simulink model "thesis_DLF_V1"  (R2024b)
settings: Solver=VariableStepAuto  StartTime=0.0  StopTime=40  FixedStep=0.001  RelTol=1e-3  EnableMultiTasking=on
undefined symbols (not defined in the file or in its folder): omega_0, p0, R0, v0
settings Model: Creator=bojack  LastModifiedBy=valer

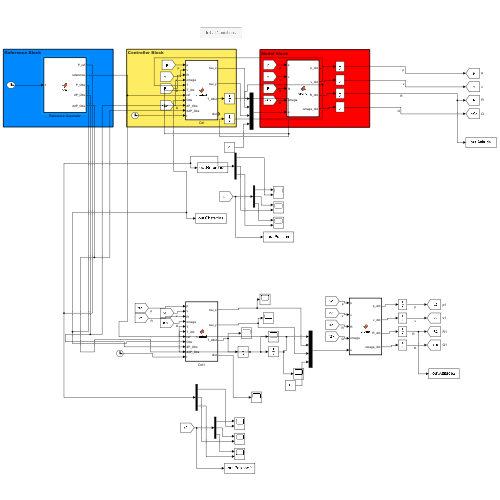
[thumbnail: Simulink's stored preview of the top-level diagram]
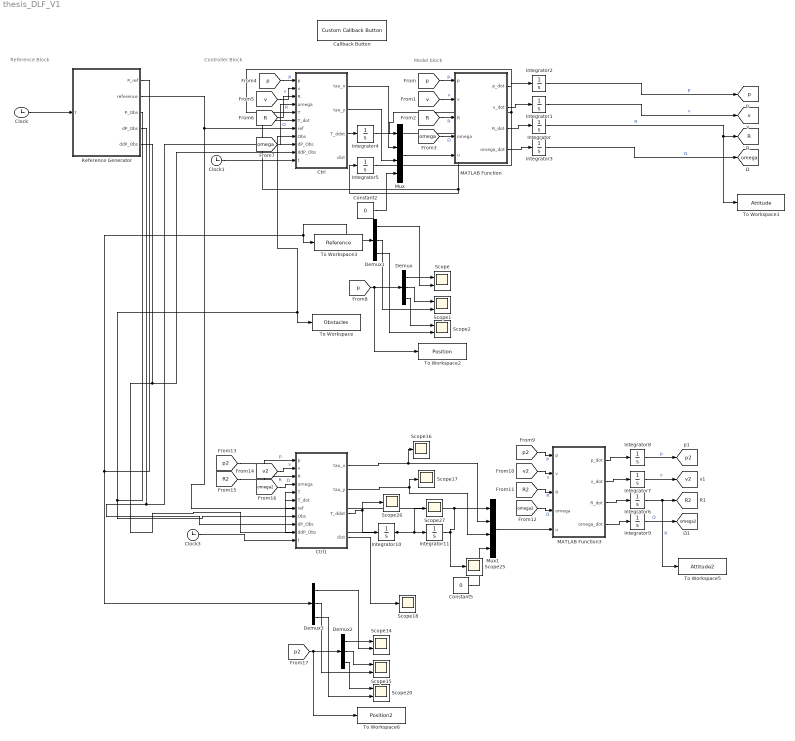
== system thesis_DLF_V1 ==
  note: Reference Block
  note: Controller Block
  note: Model block
  Callback Button : CustomCallbackButton  Configuration="{\"components\":[{\"name\":\"BackgroundImageComponent\",\"settings\":{\"image\":{\"size\":[0,0],\"src\":\"default\",\"srcOrientation\":\"Right\"},\"position\":[0,0,1,1]}},{\"name\":\"ButtonStateComponent\",\"settings\":{\"buttonType\":\"momentary\",\"clickFcn\":\"p0 = [10 0 0]';\\nv0 = [-0.5 4.5 1]';\\nR0 = eye(3);\\n\\nomega_0 = [0 0 0]';\",\"onValue\":1,\"position\":[0,0,1,1],\"pressDelay\":\"500\",\"pressFcn\":\"\",\"repeatInterval\":\"0\",\"states\":[{\"horizontalAlignment\":\"center\",\"image\":{\"position\":[0,0,1,1],\"size\":[1,1],\"src\":\"default\",\"srcOrientation\":\"Right\"},\"label\":{\"color\":[0.01176470588,0.01176470588,0.01176470588,1],\"icon\":{\"size\":[0,0],\"src\":\"default\",\"srcOrientation\":\"Right\"},\"iconOffset\":0,\"iconPlacement\":\"left\",\"opacity\":1,\"show\":true,\"text\":{\"content\":\"Initial Conditions\",\"font\":\"Helvetica\"}},\"labelOffset\":[0,0],\"verticalAlignment\":\"middle\"},{\"horizontalAlignment\":\"center\",\"image\":{\"position\":[0,0,1,1],\"size\":[1,1],\"src\":\"default\",\"srcOrientation\":\"Right\"},\"label\":{\"color\":[0.01176470588,0.01176470588,0.01176470588,1],\"icon\":{\"size\":[0,0],\"src\":\"default\",\"srcOrientation\":\"Right\"},\"iconOffset\":0,\"iconPlacement\":\"left\",\"opacity\":1,\"show\":true,\"text\":{\"content\":\"Initial Conditions\",\"font\":\"Helvetica\"}},\"labelOffset\":[0,0],\"verticalAlignment\":\"middle\"},{\"horizontalAlignment\":\"center\",\"image\":{\"position\":[0,0,1,1],\"size\":[1,1],\"src\":\"default\",\"srcOrientation\":\"Right\"},\"label\":{\"color\":[0.01176470588,0.01176470588,0.01176470588,1],\"icon\":{\"size\":[0,0],\"src\":\"default\",\"srcOrientation\":\"Right\"},\"iconOffset\":0,\"iconPlacement\":\"left\",\"opacity\":1,\"show\":true,\"text\":{\"content\":\"Initial Conditions\",\"font\":\"Helvetica\"}},\"labelOffset\":[0,0],\"verticalAlignment\":\"middle\"},{\"horizontalAlignment\":\"center\",\"image\":{\"position\":[0,0,1,1],\"size\":[1,1],\"src\":\"default\",\"srcOrientation\":\"Right\"},\"label\":{\"color\":[0.01176470588,0.01176470588,0.01176470588,1],\"icon\":{\"size\":[0,0],\"src\":\"default\",\"srcOrientation\":\"Right\"},\"iconOffset\":0,\"iconPlacement\":\"left\",\"opacity\":1,\"show\":true,\"text\":{\"content\":\"Initial Conditions\",\"font\":\"Helvetica\"}},\"labelOffset\":[0,0],\"verticalAlignment\":\"middle\"}]}},{\"name\":\"ForegroundImageComponent\",\"settings\":{\"image\":{\"size\":[0,0],\"src\":\"default\",\"srcOrientation\":\"Right\"},\"isForeground\":1,\"position\":[0,0,1,1]}}],\"settings\":{\"BindingType\":\"standalone\",\"backgroundColor\":[244,244,244,1],\"backgroundOffset\":0.2,\"backgroundOpacity\":1,\"fixedAspectRatio\":\"off\",\"foregroundColor\":[0.01176470588,0.01176470588,0.01176470588,1],\"migratedFromLegacy\":true,\"useBackgroundColor\":true,\"variant\":\"callback\",\"version\":\"R2023a\"},\"type\":\"Button\"}"  CustomBackgroundColor="{\"color\":[0.9568627450980393,0.9568627450980393,0.9568627450980393],\"show\":true}"
  Clock : Clock
  Clock1 : Clock
  Clock3 : Clock
  Constant2 : Constant  Value=0
  Constant5 : Constant  Value=0
  Ctrl : MATLAB Function  TreatAsAtomicUnit=on
  Ctrl1 : MATLAB Function  TreatAsAtomicUnit=on
  Demux{,1..3} (4 alike) : Demux  Outputs=3
  Integrator : Integrator  InitialCondition=R0
  Integrator1 : Integrator  InitialCondition=v0
  Integrator10 : Integrator  UpperSaturationLimit=0  LowerSaturationLimit=-10^6
  Integrator11 : Integrator  InitialCondition=9.81  UpperSaturationLimit=1000  LowerSaturationLimit=-1000
  Integrator2 : Integrator  InitialCondition=p0
  Integrator3 : Integrator  InitialCondition=omega_0
  Integrator4 : Integrator  UpperSaturationLimit=0  LowerSaturationLimit=-10^6
  Integrator5 : Integrator  InitialCondition=9.81  UpperSaturationLimit=1000  LowerSaturationLimit=-1000
  Integrator6 : Integrator  InitialCondition=R0
  Integrator7 : Integrator  InitialCondition=v0
  Integrator8 : Integrator  InitialCondition=p0
  Integrator9 : Integrator  InitialCondition=omega_0
  MATLAB Function : MATLAB Function  TreatAsAtomicUnit=on
  MATLAB Function3 : MATLAB Function  TreatAsAtomicUnit=on
  Mux : Mux
  Mux1 : Mux
  Reference Generator : MATLAB Function  TreatAsAtomicUnit=on
  Scope{,1..2,14..15,20} (6 alike) : Scope  NumInputPorts=2
  Scope{16..18,25..27} (6 alike) : Scope
  To Workspace : ToWorkspace  VariableName=Obstacles  SaveFormat=Structure With Time  SampleTime=0.1
  To Workspace1 : ToWorkspace  VariableName=Attitude  SaveFormat=Structure With Time  SampleTime=0.1
  To Workspace2 : ToWorkspace  VariableName=Position  SaveFormat=Structure With Time  SampleTime=0.1
  To Workspace3 : ToWorkspace  VariableName=Reference  SaveFormat=Structure With Time  SampleTime=0.1
  To Workspace5 : ToWorkspace  VariableName=Attitude2  SaveFormat=Structure With Time  SampleTime=0.1
  To Workspace6 : ToWorkspace  VariableName=Position2  SaveFormat=Structure With Time  SampleTime=0.1
  tag scope: R2=global, R=global, omega2=global, omega=global, p2=global, p=global, v2=global, v=global
  wires:
  MATLAB Function/3(R_dot) -> Integrator/1
  MATLAB Function/2(v_dot) -> Integrator1/1
  MATLAB Function/1(p_dot) -> Integrator2/1
  Integrator/1 -> To Workspace1/1, [R]  "R"
  Integrator1/1 -> [v]  "v"
  Integrator2/1 -> [p]  "p"
  MATLAB Function/4(omega_dot) -> Integrator3/1
  Integrator3/1 -> [omega]  "Ω"
  [p] -> MATLAB Function/1(p)  "p"
  [v] -> MATLAB Function/2(v)  "v"
  [R] -> MATLAB Function/3(R)  "R"
  [omega] -> MATLAB Function/4(omega)  "Ω"
  Demux/1 -> Scope/1
  Demux/2 -> Scope1/1
  Demux/3 -> Scope2/1
  [omega] -> Ctrl/4(omega)  "Ω"
  [v] -> Ctrl/2(v)  "v"
  [p] -> Ctrl/1(p)  "p"
  Ctrl/3(T_ddot) -> Integrator4/1
  Integrator4/1 -> Ctrl/6(T_dot), Integrator5/1
  Integrator5/1 -> Mux/1, Ctrl/5(T)
  Clock/1 -> Reference Generator/1(t)
  Reference Generator/2(reference) -> Ctrl1/7(ref), Ctrl/7(ref)
  [R] -> Ctrl/3(R)  "R"
  Constant2/1 -> Mux/4
  Mux/1 -> MATLAB Function/5(u)
  [p] -> To Workspace2/1, Demux/1
  Reference Generator/1(P_ref) -> Demux1/1, To Workspace3/1, Demux3/1
  Demux1/1 -> Scope/2
  Demux1/2 -> Scope1/2
  Demux1/3 -> Scope2/2
  Reference Generator/3(P_Obs) -> Ctrl1/8(Obs), Ctrl/8(Obs), To Workspace/1
  Ctrl/1(tau_x) -> Mux/2
  Ctrl/2(tau_y) -> Mux/3
  Clock1/1 -> Ctrl/11(t)
  MATLAB Function3/3(R_dot) -> Integrator6/1
  [R2] -> MATLAB Function3/3(R)  "R"
  [omega2] -> Ctrl1/4(omega)  "Ω"
  Demux2/3 -> Scope20/1
  Demux2/2 -> Scope15/1
  [v2] -> MATLAB Function3/2(v)  "v"
  [omega2] -> MATLAB Function3/4(omega)  "Ω"
  Clock3/1 -> Ctrl1/11(t)
  [p2] -> Ctrl1/1(p)  "p"
  [v2] -> Ctrl1/2(v)  "v"
  Integrator9/1 -> [omega2]  "Ω"
  [p2] -> MATLAB Function3/1(p)  "p"
  MATLAB Function3/4(omega_dot) -> Integrator9/1
  Integrator11/1 -> Mux1/1, Ctrl1/5(T), Scope25/1
  Integrator8/1 -> [p2]  "p"
  Demux2/1 -> Scope14/1
  MATLAB Function3/1(p_dot) -> Integrator8/1
  Mux1/1 -> MATLAB Function3/5(u)
  [R2] -> Ctrl1/3(R)  "R"
  [p2] -> To Workspace6/1, Demux2/1
  Ctrl1/4(dist) -> Scope18/1
  Demux3/3 -> Scope20/2
  Demux3/2 -> Scope15/2
  Integrator7/1 -> [v2]  "v"
  MATLAB Function3/2(v_dot) -> Integrator7/1
  Constant5/1 -> Mux1/4
  Ctrl1/2(tau_y) -> Scope17/1, Mux1/3
  Integrator10/1 -> Scope27/1, Integrator11/1, Ctrl1/6(T_dot)
  Ctrl1/1(tau_x) -> Scope16/1, Mux1/2
  Ctrl1/3(T_ddot) -> Scope26/1, Integrator10/1
  Demux3/1 -> Scope14/2
  Integrator6/1 -> To Workspace5/1, [R2]  "R"
  Reference Generator/4(dP_Obs) -> Ctrl1/9(dP_Obs), Ctrl/9(dP_Obs)
  Reference Generator/5(ddP_Obs) -> Ctrl1/10(ddP_Obs), Ctrl/10(ddP_Obs)

== matlab function thesis_DLF_V1/MATLAB Function ==
  data: p input; v input; p_dot output; v_dot output; R input; R_dot output; omega input; omega_dot output; u input
function [p_dot, v_dot, R_dot, omega_dot]= drone(p,v,R,omega, u)

% States
wx = omega(1);
wy = omega(2);
wz = omega(3);

% Inputs
T = u(1);
Tau = u(2:4);

% Parameters
Ix = 0.082;
Iy = 0.0845;
Iz = 0.1377;
J = diag([Ix Iy Iz]);
%J = eye(3)*0.01;%diag([Ix Iy Iz]);
g = 9.81;
m = 1;


e3 = [0 0 1]';
S = [0 -wz wy; wz 0 -wx; -wy wx 0];

% Gyroscopic effects
wx_gyro = 0;
wy_gyro = 0;

w_gyro = [wx_gyro wy_gyro 0]';
%% STATE SPACE MODEL
p_dot = v;
v_dot = -e3*g + R*e3*T/m;
R_dot = R*S;
omega_dot = J\(cross(omega,J*omega)+w_gyro+Tau);

== matlab function thesis_DLF_V1/Ctrl ==
  data: tau_x output; tau_y output; T_ddot output; p input; v input; R input; omega input; T input; T_dot input; ref input; Obs input; dP_Obs input; ddP_Obs input; t input; dist output
function [tau_x, tau_y, T_ddot, dist] = control(p,v,R,omega,T , T_dot, ref, Obs, dP_Obs, ddP_Obs, t)

M = diag([1/0.5^2 1/0.5^2 1/0.25^2]);
mu =0.5;
mu2 = 0.01;
delta = 20;
%muro
%delta =20
%mu = 0.8;
%mu2 = 0.007;
% States
wx = omega(1);
wy = omega(2);
wz = omega(3);

% Parameters
Ix = 0.082;
Iy = 0.0845;
Iz = 0.1377;
J = diag([Ix Iy Iz]);
g = 9.81;
m = 1;


e3 = [0 0 1]';
S = [0 -wz wy; wz 0 -wx; -wy wx 0];

%% Linear PID terms
p_ref = ref(:,1);
v_ref = ref(:,2);
a_ref = ref(:,3);
j_ref = ref(:,4);
dj_ref = ref(:,5);

a = -e3*g + R*e3*T/m;

j = R/m*[wy -wx 0]'*T + e3*T_dot;

% -[1     7    14     8]

VV = (1*(p_ref - p) + 7*(v_ref - v) + 14*(a_ref - a ) + 8*(j_ref - j )) + dj_ref;
VV = (24*(p_ref - p) + 50*(v_ref - v) + 35*(a_ref - a ) + 10*(j_ref - j )) + dj_ref;
%% CBF
distanza=zeros(size(Obs,1),1);

for i = 1: size(Obs,1)
    distanza(i)=norm(p-Obs(i,:)');
end
[value,index]=min(distanza);

p_obs=Obs(index,:)';
v_obs = dP_Obs(index,:)';
a_obs = ddP_Obs(index,:)';

V = p - p_obs;
V_dot = v - v_obs;
V_ddot = a - a_obs;

R_dot = R*S;
h = V'*R'*M*R*V + mu*V'*M*V_dot + mu2*V'*M*j - 1.5;
dist = sqrt(V'*V);
h_dot = 2*V'*R'*M*R*V_dot + V'*(R_dot'*M*R + R'*M*R_dot)*V + ...
    mu2*V_dot'*M*j  +...
    mu*V'*M*V_ddot + mu2*V'*M*VV;



if h > delta || h_dot > 0
u = VV;

else

proj = V*(V'*V)^-(1)*V';
proj_perp = eye(3) - proj;
M_inv = inv(M);

u = -(1/mu2)*M_inv*proj*(mu*M*V_ddot + 2*R'*M*R*V_dot + (R_dot'*M*R + R'*M*R_dot)*V) - M_inv*pinv(V')*V_dot'*M*j + ...
   M_inv*proj_perp*VV;


t
end


%T_ddot = u(3);
%{
if abs(T) < 1e-3
T = 1e-3*sign(T);
end
%}

u_bar = m*R'*u;
tau_y = Iy*(((Ix - Iz)/Iy - 1)*wx*wz - 2*wy*T_dot/T + u_bar(1)/T);
tau_x = Ix*(((Iz - Iy)/Ix + 1)*wy*wz - 2*wx*T_dot/T - u_bar(2)/T);

T_ddot = (wx^2 + wy^2)*T + u_bar(3);

== matlab function thesis_DLF_V1/Reference Generator ==
  data: t input; P_ref output; reference output; P_Obs output; dP_Obs output; ddP_Obs output
function [P_ref, reference, P_Obs, dP_Obs, ddP_Obs] = fcn(t)
w = 0.5;
x_ref= 10*cos(w*t);
y_ref= 10*sin(w*t);
z_ref= 1*t;


vx_ref= -w*10*sin(w*t);
vy_ref= w*10*cos(w*t);
vz_ref= 1;

ax_ref= -w^2*x_ref;
ay_ref= -w^2*y_ref;
az_ref= 0;

jx_ref= w^3*10*sin(w*t);
jy_ref= -w^3*10*cos(w*t);
jz_ref= 0;

djx_ref= w^4*10*cos(w*t);
djy_ref= w^4*10*sin(w*t);
djz_ref= 0;

%retta
% x_ref= 1*t;
% y_ref= 0;
% z_ref= 0;
% 
% 
% vx_ref= 1;
% vy_ref= 0;
% vz_ref= 0;
% 
% ax_ref= 0;
% ay_ref= 0;
% az_ref= 0;
% 
% jx_ref= 0;
% jy_ref= 0;
% jz_ref= 0;
% 
% djx_ref= 0;
% djy_ref= 0;
% djz_ref= 0;


%%%%  %%%%%%
P_ref= [x_ref y_ref z_ref]';
V_ref= [vx_ref vy_ref vz_ref]';
A_ref= [ax_ref ay_ref az_ref]';
J_ref= [jx_ref jy_ref jz_ref]';
dJ_ref= [djx_ref djy_ref djz_ref]';

reference = [P_ref V_ref A_ref J_ref dJ_ref];
%%%%  %%%%%%

w_obs=0.5;
P_Obs = [2.8366 -9.5892 12;
         11.5 1.908 25.5;
         8.5 1.7 25;
         8 1.8 28;
         -9 5*cos(w_obs*t) 32];
dP_Obs = [zeros(4,3);
          0 -5*w_obs*sin(w_obs*t) 0];
ddP_Obs =[zeros(4,3); 
          0 -5*w_obs^2*cos(w_obs*t) 0];

%ostacoli retta finestra
% 
% P_Obs = [20 0 -1; %[z x(sotto) y(sinistra]
%          20 2 -1;
%          19.6 0.3 1;
%          20 -1.5 -0.3;
%          20 0 3;
%          20 1 0;
%          20 2 1; 
%          20 -2.2 4; %3
%          20 -2.2 -1;
%          20 -3.3 1.5]; %-4.3
% dP_Obs = [zeros(10,3)];
% ddP_Obs =[zeros(10,3)];

== matlab function thesis_DLF_V1/Ctrl1 ==
  data: tau_x output; tau_y output; T_ddot output; p input; v input; R input; omega input; T input; T_dot input; ref input; Obs input; dP_Obs input; ddP_Obs input; t input; dist output
function [tau_x, tau_y, T_ddot, dist] = control(p,v,R,omega,T , T_dot, ref, Obs, dP_Obs, ddP_Obs, t)


mu =0.5;
mu2 = 0.01;
delta = 20;
%muro
% mu = 0.8;
% mu2 = 0.007;
% delta =5 ;
% States
wx = omega(1);
wy = omega(2);
wz = omega(3);

% Parameters
Ix = 0.082;
Iy = 0.0845;
Iz = 0.1377;
J = diag([Ix Iy Iz]);
g = 9.81;
m = 1;


e3 = [0 0 1]';
S = [0 -wz wy; wz 0 -wx; -wy wx 0];

%% Linear PID terms

p_ref = ref(:,1);
v_ref = ref(:,2);
a_ref = ref(:,3);
j_ref = ref(:,4);
dj_ref = ref(:,5);

a = -e3*g + R*e3*T/m;

j = R/m*[wy -wx 0]'*T + e3*T_dot;
% -[1     7    14     8]

VV = (1*(p_ref - p) + 7*(v_ref - v) + 14*(a_ref - a ) + 8*(j_ref - j )) + dj_ref;
VV = (24*(p_ref - p) + 50*(v_ref - v) + 35*(a_ref - a ) + 10*(j_ref - j )) + dj_ref;

%% CBF

distanza=zeros(size(Obs,1),1);

for i = 1: size(Obs,1)
    distanza(i)=norm(p-Obs(i,:)');
end
[value,index]=min(distanza);

p_obs=Obs(index,:)';
v_obs = dP_Obs(index,:)';
a_obs = ddP_Obs(index,:)';


V = p - p_obs;
V_dot = v - v_obs;
V_ddot = a - a_obs;

h = V'*V + mu*V'*V_dot + mu2*V'*j - 1.5;
dist = sqrt(V'*V);
h_dot = 2*V'*V_dot + mu2*V_dot'*j  + mu*V'*V_ddot + mu2*V'*VV;


if h > delta || h_dot > 0
u = VV;
else
proj = V*(V'*V)^-(1)*V';
proj_perp = eye(3) - proj;

u = -(1/mu2)*proj*(mu*V_ddot + 2*V_dot) - pinv(V')*V_dot'*j + proj_perp*VV;
end

u_bar = m*R'*u;

tau_y = Iy*(((Ix - Iz)/Iy - 1)*wx*wz - 2*wy*T_dot/T + u_bar(1)/T);
tau_x = Ix*(((Iz - Iy)/Ix + 1)*wy*wz - 2*wx*T_dot/T - u_bar(2)/T);

T_ddot = (wx^2 + wy^2)*T + u_bar(3);

== matlab function thesis_DLF_V1/MATLAB Function3 ==
  data: p input; v input; p_dot output; v_dot output; R input; R_dot output; omega input; omega_dot output; u input
function [p_dot, v_dot, R_dot, omega_dot]= drone(p,v,R,omega, u)

% States
wx = omega(1);
wy = omega(2);
wz = omega(3);

% Inputs
T = u(1);
Tau = u(2:4);

% Parameters
Ix = 0.082;
Iy = 0.0845;
Iz = 0.1377;
J = diag([Ix Iy Iz]);
%J = eye(3)*0.01;%diag([Ix Iy Iz]);
g = 9.81;
m = 1;


e3 = [0 0 1]';
S = [0 -wz wy; wz 0 -wx; -wy wx 0];

% Gyroscopic effects
wx_gyro = 0;
wy_gyro = 0;

w_gyro = [wx_gyro wy_gyro 0]';
%% STATE SPACE MODEL
p_dot = v;
v_dot = -e3*g + R*e3*T/m;
R_dot = R*S;
omega_dot = J\(cross(omega,J*omega)+w_gyro+Tau);
